simulink model "pacing_unit"  (R2023b)
settings: Solver=FixedStepAuto  StartTime=0.0  StopTime=10.0  FixedStep=1e-3  RelTol=1e-3  EnableMultiTasking=on
undefined symbols (not defined in the file): D8, PTA0
libraries: frdmk64flib x1
settings Model: ExtModeTrigDuration=5  Creator=haley  LastModifiedBy=haley
settings OptimizationCC: EnhancedBackFolding=on  PassReuseOutputArgsAs=Individual arguments  ZeroExternalMemoryAtStartup=off  ZeroInternalMemoryAtStartup=off  MaxStackSize=64  OptimizeBlockOrder=speed  DifferentSizesBufferReuse=on  OptimizationCustomize=off  EfficientTunableParamExpr=on
settings DebuggingCC: ParameterTunabilityLossMsg=error
settings HardwareCC: ProdBitPerPointer=32  ProdBitPerSizeT=32  ProdBitPerPtrDiffT=32  ProdLargestAtomicInteger=Long  ProdLargestAtomicFloat=Double  ProdWordSize=32  ProdHWDeviceType=ARM Compatible->ARM Cortex
settings SFSimCC: MATLABDynamicMemAlloc=off
settings RTWCC: Description=Embedded Coder  SystemTargetFile=ert.tlc  HardwareBoard=NXP FRDM-K64F  TLCOptions="-aInlineSetEventsForThisBaseRateFcn=TLC_FALSE -aSuppressMultiTaskScheduler=TLC_FALSE  -aRateBasedStepFcn=0"  TemplateMakefile=ert_default_tmf  Toolchain=GNU Tools for ARM Embedded Processors
settings CodeAppCC: ForceParamTrailComments=on  IgnoreCustomStorageClasses=off  OperatorAnnotations=on  SimulinkDataObjDesc=on  SFDataObjDesc=on  InsertBlockDesc=on
settings ERTTargetCC: ExtModeTransport=4  ExtModeMexFile=sendToCommService

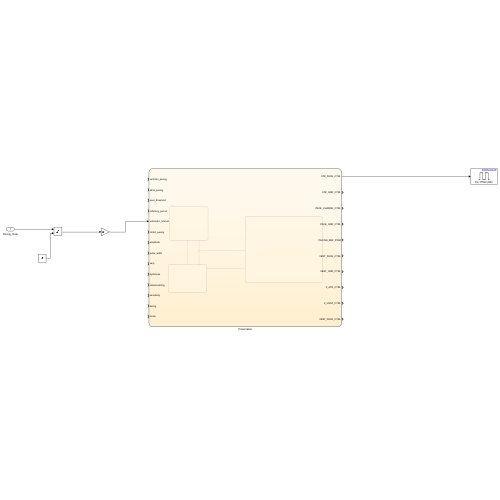
[thumbnail: Simulink's stored preview of the top-level diagram]
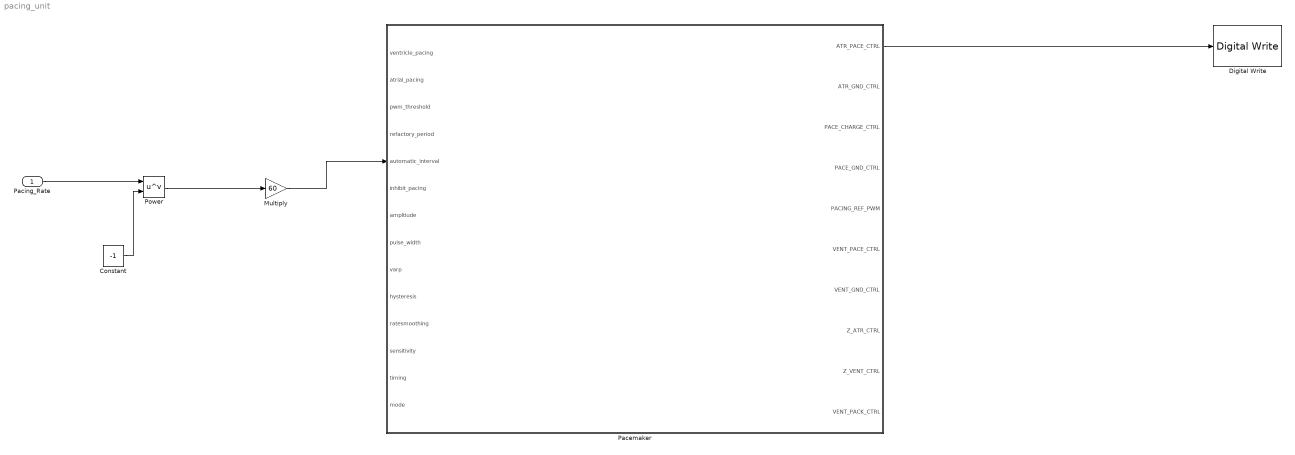
== system pacing_unit ==
  Pacing_Rate : Inport
  Constant : Constant  Value=-1
  Digital Write : frdmk64flib/Digital Write  Whichpin=PTA0 (D8)
  Multiply : Gain  Gain=60
  Pacemaker : Stateflow chart  TreatAsAtomicUnit=on
  Power : Math  Operator=pow
  wires:
  Pacemaker/1(ATR_PACE_CTRL) -> Digital Write/1
  Power/1 -> Multiply/1
  Multiply/1 -> Pacemaker/5(automatic_interval)
  Constant/1 -> Power/2
  Pacing_Rate/1 -> Power/1

== stateflow chart pacing_unit/Pacemaker ==
  state Charge_Discharge_C22
    entry:
    %Charge
    ATR_PACE_CTRL = 0;
    VENT_PACE_CTRL = 0;
    PACE_CHARGE_CTRL = 1;
    PACING_REF_PWM = pwm_threshold; %percentage
    %Discharge
    PACE_GND_CTRL = 1;
    VENT_PACK_CTRL = 0;
    Z_ATR_CTRL = 0;
    Z_VENT_CTRL = 0;
    ATR_PACE_CTRL = 0;
    ATR_GND_CTRL = atrial_pacing;
    VENT_GND_CTRL= ventricle_pacing;
  state Sensing
  state ChargeC21
    %Creates the leading edge and sends pulse for X amount of time
    entry:
    PACE_CHARGE_CTRL = 0;
    PACE_GND_CTRL = 1;
    ATR_PACE_CTRL = atrial_pacing;
    ATR_GND_CTRL = 0;
    Z_ATR_CTRL = 0;
    Z_VENT_CTRL = 0;
    VENT_GND_CTRL = 0;
    VENT_PACE_CTRL = ventricle_pacing;
    %Recharge pulse is the current in the opposite direction due to C21
  (default) -> Charge_Discharge_C22
  ChargeC21 -> Charge_Discharge_C22 : after(pulse_width, sec)
  Charge_Discharge_C22 -> (junction 67) : after(refactory_period, sec)
  (junction 67) -> Sensing [order 1] : [mode == 1]
  (junction 67) -> ChargeC21 [order 2] : [mode == 0 && after(automatic_interval, sec)]
  Sensing -> ChargeC21 : %statement where the timer has elasped
  data: ventricle_pacing input; atrial_pacing input; pwm_threshold input; ATR_PACE_CTRL output; ATR_GND_CTRL output; PACE_CHARGE_CTRL output; PACE_GND_CTRL output; PACING_REF_PWM output; VENT_PACE_CTRL output; VENT_GND_CTRL output; Z_ATR_CTRL output; Z_VENT_CTRL output; refactory_period input; automatic_interval input; inhibit_pacing input; ampltiude input; pulse_width input; varp input; hysteresis input; ratesmoothing input; sensitivity input; timing input; mode input; VENT_PACK_CTRL output
